simulink model "sun_vector_test"  (R2016b)
settings: Solver=VariableStepAuto  StartTime=0.0  StopTime=86400  RelTol=1e-3
undefined symbols (not defined in the file): fsw_params
libraries: environment_lib x1, time_conversions_lib x1, sgp4_lib_fsw x1, sun_vector_lib x1, teme_2_eci_lib x1
settings Model: Creator=Taylor  LastModifiedBy=Taylor

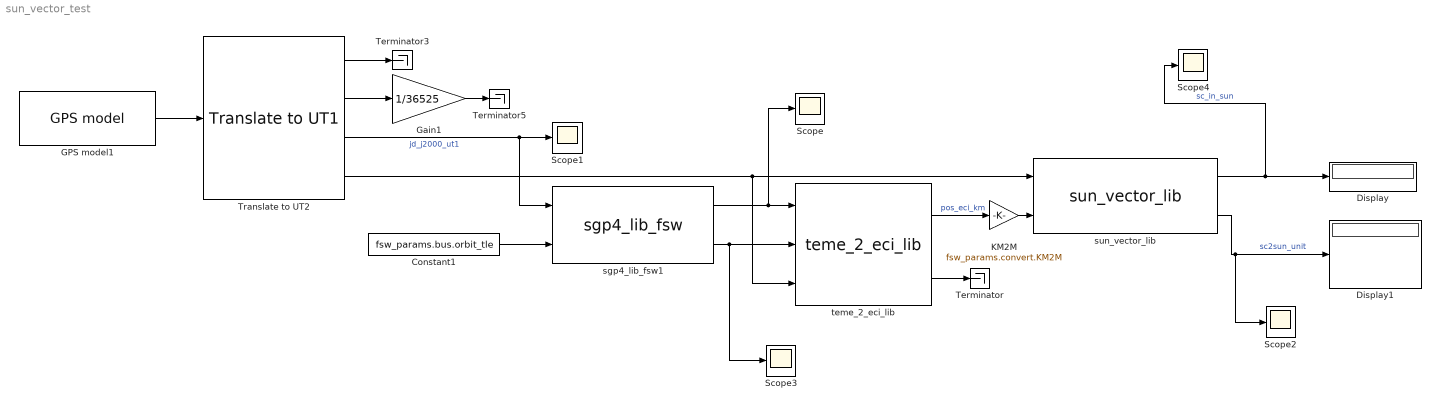
== system sun_vector_test ==
  Constant1 : Constant  Value=fsw_params.bus.orbit_tle
  Display : Display
  Display1 : Display
  GPS model1 : environment_lib/Environment/GPS model
  Gain1 : Gain  Gain=1/36525
  KM2M : Gain  Gain=fsw_params.convert.KM2M
  Scope{,1..4} (5 alike) : Scope
  Terminator : Terminator
  Terminator3 : Terminator
  Terminator5 : Terminator
  Translate to UT2 : time_conversions_lib/Translate to UT1
  sgp4_lib_fsw1 : sgp4_lib_fsw/sgp4_lib_fsw
  sun_vector_lib : sun_vector_lib/sun_vector_lib
  teme_2_eci_lib : teme_2_eci_lib/teme_2_eci_lib
  wires:
  sun_vector_lib/1 -> Scope4/1, Display/1  "sc_in_sun"
  sun_vector_lib/2 -> Scope2/1, Display1/1  "sc2sun_unit"
  sgp4_lib_fsw1/1 -> Scope/1, teme_2_eci_lib/1
  sgp4_lib_fsw1/2 -> Scope3/1, teme_2_eci_lib/2
  teme_2_eci_lib/1 -> KM2M/1  "pos_eci_km"
  teme_2_eci_lib/2 -> Terminator/1
  Translate to UT2/3 -> Scope1/1, sgp4_lib_fsw1/1  "jd_j2000_ut1"
  Translate to UT2/4 -> teme_2_eci_lib/3, sun_vector_lib/1
  Constant1/1 -> sgp4_lib_fsw1/2
  KM2M/1 -> sun_vector_lib/2
  GPS model1/1 -> Translate to UT2/1
  Translate to UT2/2 -> Gain1/1
  Translate to UT2/1 -> Terminator3/1
  Gain1/1 -> Terminator5/1
